simulink model "stateEstimator"  (R2018a)
settings: Solver=VariableStepAuto  StartTime=0.0  StopTime=10.0  RelTol=1e-3
undefined symbols (not defined in the file): SkywalkerX8
libraries: simulink_extras x5, sharedTrackingLibrary x2
settings Model: Creator=David  LastModifiedBy=David

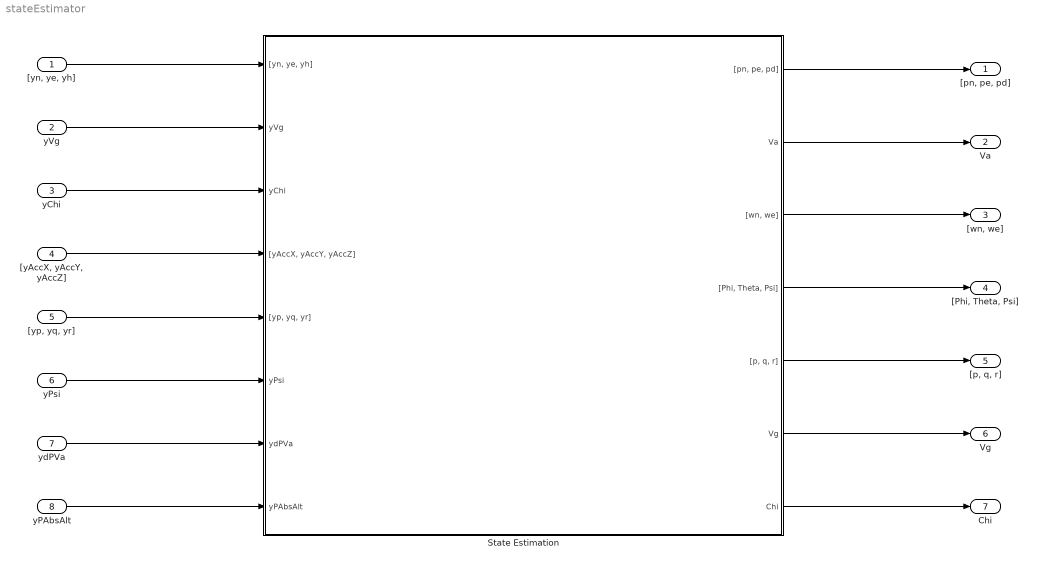
== system stateEstimator ==
  "[yn, ye, yh]" : Inport  PortDimensions=3
  yVg : Inport  Port=2  PortDimensions=3
  yChi : Inport  Port=3  PortDimensions=3
  "[yAccX, yAccY, yAccZ]" : Inport  Port=4  PortDimensions=3
  "[yp, yq, yr]" : Inport  Port=5  PortDimensions=3
  yPsi : Inport  Port=6  PortDimensions=3
  ydPVa : Inport  Port=7  PortDimensions=3
  yPAbsAlt : Inport  Port=8  PortDimensions=3
  State Estimation : Subsystem
      mask Display:
      | image('state_estimate.jpg', 'center')
      | 
      | port_label('input', 1, '[y_{GPS_N}, y_{GPS_E}, y_{GPS_h}] (m)', 'texMode', 'On')
      | port_label('input', 2, 'y_{GPS_{Vg}} (m/s)', 'texMode', 'On')
      | port_label('input', 3, 'y_{GPS_{\chi}} (rad)', 'texMode', 'On')
      | port_label('input', 4, '[y_{accel_x}, y_{accel_y}, y_{accel_z}] (m/s^2)', 'texMode', 'on')
      | port_label('input', 5, '[y_p, y_q, y_r] (rad/s)', 'texMode', 'on')
      | port_label('input', 6, 'y_{\psi} (rad)', 'texMode', 'on')
      | port_label('input', 7, 'y_{\DeltaP_{V_a}} (Pa)', 'texMode', 'on')
      | port_label('input', 8, 'y_{P_{abs}} (Pa)', 'texMode', 'on')
      | 
      | port_label('output', 1, '[p_N, p_E, p_D] (m)', 'texMode', 'On')
      | port_label('output', 2, 'V_a (m/s)', 'texMode', 'On')
      | port_label('output', 3, '[w_N, w_E] (m/s)', 'texMode', 'On')
      | port_label('output', 4, '[\phi, \theta, \psi] (rad)', 'texMode', 'on')
      | port_label('output', 5, '{\bf\omega_b} (rad/s)', 'texMode', 'on')
      | port_label('output', 6, 'V_g (m/s)', 'texMode', 'on')
      | port_label('output', 7, '\chi (rad)', 'texMode', 'on')
  "[pn, pe, pd]" : Outport
  Va : Outport  Port=2
  "[wn, we]" : Outport  Port=3
  "[Phi, Theta, Psi]" : Outport  Port=4
  "[p, q, r]" : Outport  Port=5
  Vg : Outport  Port=6
  Chi : Outport  Port=7
  wires:
  "[yn, ye, yh]"/1 -> State Estimation/1("[yn, ye, yh]")
  yVg/1 -> State Estimation/2(yVg)
  yChi/1 -> State Estimation/3(yChi)
  "[yAccX, yAccY, yAccZ]"/1 -> State Estimation/4("[yAccX, yAccY, yAccZ]")
  "[yp, yq, yr]"/1 -> State Estimation/5("[yp, yq, yr]")
  yPsi/1 -> State Estimation/6(yPsi)
  ydPVa/1 -> State Estimation/7(ydPVa)
  yPAbsAlt/1 -> State Estimation/8(yPAbsAlt)
  State Estimation/1("[pn, pe, pd]") -> "[pn, pe, pd]"/1
  State Estimation/2(Va) -> Va/1
  State Estimation/3("[wn, we]") -> "[wn, we]"/1
  State Estimation/4("[Phi, Theta, Psi]") -> "[Phi, Theta, Psi]"/1
  State Estimation/5("[p, q, r]") -> "[p, q, r]"/1
  State Estimation/6(Vg) -> Vg/1
  State Estimation/7(Chi) -> Chi/1

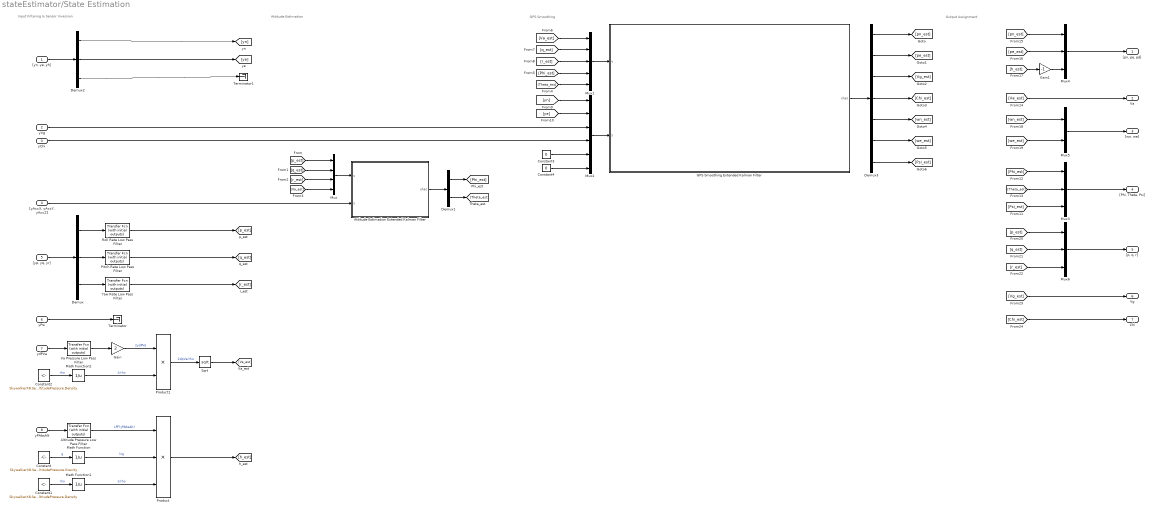
== system stateEstimator/State Estimation ==
  note: Output Assignment
  note: GPS Smoothing
  note: Attitude Estimation
  note: Input Filtering & Sensor Inversion
  "[yn, ye, yh]" : Inport  PortDimensions=3
  yVg : Inport  Port=2  PortDimensions=3
  yChi : Inport  Port=3  PortDimensions=3
  "[yAccX, yAccY, yAccZ]" : Inport  Port=4  PortDimensions=3
  "[yp, yq, yr]" : Inport  Port=5  PortDimensions=3
  yPsi : Inport  Port=6  PortDimensions=3
  ydPVa : Inport  Port=7  PortDimensions=3
  yPAbsAlt : Inport  Port=8  PortDimensions=3
  Altitude Pressure Low Pass Filter : simulink_extras/Additional Linear/Transfer Fcn (with initial outputs)  N=cell2mat(SkywalkerX8.Sensors.Filters.AltitudePressure.FilterTF.Numerator)  D=cell2mat(SkywalkerX8.Sensors.Filters.AltitudePressure.FilterTF.Denominator)  Y0=SkywalkerX8.Sensors.Filters.AltitudePressure.InitialCondition  U0=SkywalkerX8.Sensors.Filters.AltitudePressure.InitialCondition
  Attitude Estimation Extended Kalman Filter : Subsystem
      mask Display:
      | port_label('input', 1, '{\bf u} = [p, q, r, V_a]', 'texMode', 'On')
      | port_label('input', 2, '{\bf y} = [a_x, a_y, a_z]', 'texMode', 'On')
      | 
      | port_label('output', 1, '{\bf x_{est}} = [\Phi, \theta]', 'texMode', 'On')
  Constant : Constant  Value=SkywalkerX8.Sensors.StateEstimate.SensorInversion.AltitudePressure.Gravity
  Constant1 : Constant  Value=SkywalkerX8.Sensors.StateEstimate.SensorInversion.AltitudePressure.Density
  Constant2 : Constant  Value=SkywalkerX8.Sensors.StateEstimate.SensorInversion.AltitudePressure.Density
  Constant3 : Constant  Value=0
  Constant4 : Constant  Value=0
  Demux : Demux  Outputs=3
  Demux1 : Demux  Outputs=2
  Demux2 : Demux  Outputs=3
  Demux3 : Demux  Outputs=7
  GPS Smoothing Extended Kalman Filter : Subsystem
      mask Display:
      | port_label('input', 1, '{\bf u} = [V_a, q, r, \Phi, \theta]', 'texMode', 'On')
      | port_label('input', 2, '{\bf y} = [y_{GPS_N}, y_{GPS_E}, y_{GPS_{V_g}}, y_{GPS_\chi}, y_{GPS_{wind_N}}, y_{GPS_{wind_E}}]', 'texMode', 'On')
      | 
      | port_label('output', 1, '{\bf x_{est}} = [p_n, p_e, V_g, \chi, w_n, w_e, \psi]', 'texMode', 'On')
  Gain : Gain  Gain=2
  Gain1 : Gain  Gain=-1
  Math Function : Math  Operator=reciprocal  SaturateOnIntegerOverflow=on
  Math Function1 : Math  Operator=reciprocal  SaturateOnIntegerOverflow=on
  Math Function2 : Math  Operator=reciprocal  SaturateOnIntegerOverflow=on
  Mux : Mux
  Mux1 : Mux  Inputs=5
  Mux2 : Mux  Inputs=6
  Mux3 : Mux  Inputs=3
  Mux4 : Mux  Inputs=3
  Mux5 : Mux  Inputs=2
  Mux6 : Mux  Inputs=3
  Pitch Rate Low Pass Filter : simulink_extras/Additional Linear/Transfer Fcn (with initial outputs)  N=cell2mat(SkywalkerX8.Sensors.Filters.AngularRates.Pitch.FilterTF.Numerator)  D=cell2mat(SkywalkerX8.Sensors.Filters.AngularRates.Pitch.FilterTF.Denominator)  Y0=SkywalkerX8.Sensors.Filters.AngularRates.Pitch.InitialCondition  U0=SkywalkerX8.Sensors.Filters.AngularRates.Pitch.InitialCondition
  Product : Product  Inputs=3
  Product1 : Product
  Roll Rate Low Pass Filter : simulink_extras/Additional Linear/Transfer Fcn (with initial outputs)  N=cell2mat(SkywalkerX8.Sensors.Filters.AngularRates.Roll.FilterTF.Numerator)  D=cell2mat(SkywalkerX8.Sensors.Filters.AngularRates.Roll.FilterTF.Denominator)  Y0=SkywalkerX8.Sensors.Filters.AngularRates.Roll.InitialCondition  U0=SkywalkerX8.Sensors.Filters.AngularRates.Roll.InitialCondition
  Sqrt : Sqrt  SaturateOnIntegerOverflow=on
  Terminator : Terminator
  Terminator1 : Terminator
  Va Pressure Low Pass Filter : simulink_extras/Additional Linear/Transfer Fcn (with initial outputs)  N=cell2mat(SkywalkerX8.Sensors.Filters.AirspeedPressure.FilterTF.Numerator)  D=cell2mat(SkywalkerX8.Sensors.Filters.AirspeedPressure.FilterTF.Denominator)  Y0=SkywalkerX8.Sensors.Filters.AirspeedPressure.InitialCondition  U0=SkywalkerX8.Sensors.Filters.AirspeedPressure.InitialCondition
  Yaw Rate Low Pass Filter : simulink_extras/Additional Linear/Transfer Fcn (with initial outputs)  N=cell2mat(SkywalkerX8.Sensors.Filters.AngularRates.Yaw.FilterTF.Numerator)  D=cell2mat(SkywalkerX8.Sensors.Filters.AngularRates.Yaw.FilterTF.Denominator)  Y0=SkywalkerX8.Sensors.Filters.AngularRates.Yaw.InitialCondition  U0=SkywalkerX8.Sensors.Filters.AngularRates.Yaw.InitialCondition
  "[pn, pe, pd]" : Outport
  Va : Outport  Port=2
  "[wn, we]" : Outport  Port=3
  "[Phi, Theta, Psi]" : Outport  Port=4
  "[p, q, r]" : Outport  Port=5
  Vg : Outport  Port=6
  Chi : Outport  Port=7
  wires:
  [Phi_est] -> Mux1/4
  Math Function1/1 -> Product/3  "1/rho"
  [ye] -> Mux2/2
  Sqrt/1 -> [Va_est]
  Demux/2 -> Pitch Rate Low Pass Filter/1
  [r_est] -> Mux/3
  Math Function2/1 -> Product1/2  "1/rho"
  yChi/1 -> Mux2/4
  Demux2/3 -> Terminator1/1
  Mux4/1 -> "[pn, pe, pd]"/1
  Mux6/1 -> "[p, q, r]"/1
  [r_est] -> Mux1/3
  Constant3/1 -> Mux2/5
  Constant2/1 -> Math Function2/1  "rho"
  Demux3/4 -> [Chi_est]
  Demux3/3 -> [Vg_est]
  Gain1/1 -> Mux4/3
  Math Function/1 -> Product/2  "1/g"
  [h_est] -> Gain1/1
  [we_est] -> Mux5/2
  "[yp, yq, yr]"/1 -> Demux/1
  [Theta_est] -> Mux1/5
  Demux3/7 -> [Psi_est]
  Mux2/1 -> GPS Smoothing Extended Kalman Filter/2(y)
  Constant4/1 -> Mux2/6
  [r_est] -> Mux6/3
  Mux/1 -> Attitude Estimation Extended Kalman Filter/1(u)
  [wn_est] -> Mux5/1
  Demux2/2 -> [ye]
  GPS Smoothing Extended Kalman Filter/1(xhat) -> Demux3/1
  Constant1/1 -> Math Function1/1  "rho"
  Demux2/1 -> [yn]
  Demux3/6 -> [we_est]
  [q_est] -> Mux6/2
  "[yAccX, yAccY, yAccZ]"/1 -> Attitude Estimation Extended Kalman Filter/2(y)
  Demux1/2 -> [Theta_est]
  Mux1/1 -> GPS Smoothing Extended Kalman Filter/1(u)
  Demux3/5 -> [wn_est]
  Attitude Estimation Extended Kalman Filter/1(xhat) -> Demux1/1
  Gain/1 -> Product1/1  "2ydPVa"
  Constant/1 -> Math Function/1  "g"
  [p_est] -> Mux/1
  yVg/1 -> Mux2/3
  Altitude Pressure Low Pass Filter/1 -> Product/1  "LPF(yPAbsAlt)"
  [Chi_est] -> Chi/1
  yPsi/1 -> Terminator/1
  [q_est] -> Mux1/2
  Demux3/1 -> [pn_est]
  [Va_est] -> Mux1/1
  [Theta_est] -> Mux3/2
  Va Pressure Low Pass Filter/1 -> Gain/1
  [q_est] -> Mux/2
  Product1/1 -> Sqrt/1  "2dpVa/rho"
  Yaw Rate Low Pass Filter/1 -> [r_est]
  Product/1 -> [h_est]
  [Va_est] -> Mux/4
  ydPVa/1 -> Va Pressure Low Pass Filter/1
  [Psi_est] -> Mux3/3
  Pitch Rate Low Pass Filter/1 -> [q_est]
  Demux/1 -> Roll Rate Low Pass Filter/1
  yPAbsAlt/1 -> Altitude Pressure Low Pass Filter/1
  Demux/3 -> Yaw Rate Low Pass Filter/1
  [pn_est] -> Mux4/1
  [p_est] -> Mux6/1
  Demux3/2 -> [pe_est]
  Demux1/1 -> [Phi_est]
  Roll Rate Low Pass Filter/1 -> [p_est]
  [Vg_est] -> Vg/1
  "[yn, ye, yh]"/1 -> Demux2/1
  [pe_est] -> Mux4/2
  [Phi_est] -> Mux3/1
  Mux3/1 -> "[Phi, Theta, Psi]"/1
  Mux5/1 -> "[wn, we]"/1
  [Va_est] -> Va/1
  [yn] -> Mux2/1

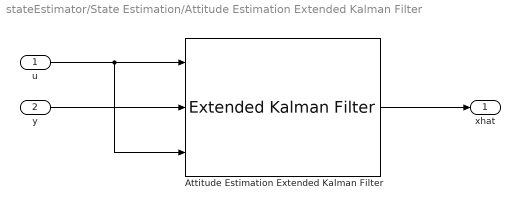
== system stateEstimator/State Estimation/Attitude Estimation Extended Kalman Filter ==
  u : Inport
  y : Inport  Port=2
  Attitude Estimation Extended Kalman Filter : sharedTrackingLibrary/Extended Kalman Filter  StateTransitionFcn=attitudeTransitionEstimate  HasStateTransitionJacobianFcn=on  StateTransitionJacobianFcn=attitudeTransitionEstimate_Jacobian  HasAdditiveProcessNoise=Additive  ProcessNoise=SkywalkerX8.Sensors.EKF.Attitude.StateCovarianceMatrix  HasTimeVaryingProcessNoise=off  HasStateTransitionFcnExtraArgument=1  InitialState=SkywalkerX8.Sensors.EKF.Attitude.InitialState  InitialStateCovariance=SkywalkerX8.Sensors.EKF.Attitude.InitialStateCovarianceMatrix  MeasurementFcn1=accelerometerMeasurementEstimate  HasMeasurementJacobianFcn1=on  MeasurementJacobianFcn1=accelerometerMeasurementEstimate_Jacobian  HasMeasurementEnablePort1=off  HasAdditiveMeasurementNoise1=Additive  MeasurementNoise1=SkywalkerX8.Sensors.EKF.Attitude.MeasurementCovarianceMatrix  HasTimeVaryingMeasurementNoise1=off  HasMeasurementFcnExtraArgument1=1  MeasurementFcn2=myMeasurementFcn  HasMeasurementJacobianFcn2=off  HasMeasurementEnablePort2=off  HasAdditiveMeasurementNoise2=Additive  MeasurementNoise2=1  HasTimeVaryingMeasurementNoise2=off  HasMeasurementFcnExtraArgument2=0  MeasurementFcn3=myMeasurementFcn  HasMeasurementJacobianFcn3=off  HasMeasurementEnablePort3=off  HasAdditiveMeasurementNoise3=Additive  MeasurementNoise3=1  HasTimeVaryingMeasurementNoise3=off  HasMeasurementFcnExtraArgument3=0  MeasurementFcn4=myMeasurementFcn  HasMeasurementJacobianFcn4=off  HasMeasurementEnablePort4=off  HasAdditiveMeasurementNoise4=Additive  MeasurementNoise4=1  HasTimeVaryingMeasurementNoise4=off  HasMeasurementFcnExtraArgument4=0  MeasurementFcn5=myMeasurementFcn  HasMeasurementJacobianFcn5=off  HasMeasurementEnablePort5=off  HasAdditiveMeasurementNoise5=Additive  MeasurementNoise5=1  HasTimeVaryingMeasurementNoise5=off  HasMeasurementFcnExtraArgument5=0  EnableMultirate=on  StateTransitionFcnSampleTime=SkywalkerX8.Sensors.EKF.Attitude.StateTransitionSampleTime  MeasurementFcn1SampleTime=SkywalkerX8.Sensors.EKF.Attitude.MeasurementSampleTime  MeasurementFcn2SampleTime=1  MeasurementFcn3SampleTime=1  MeasurementFcn4SampleTime=1  MeasurementFcn5SampleTime=1  UseCurrentEstimator=on  OutputStateCovariance=off  DataType=double  SampleTime=SkywalkerX8.Sensors.EKF.Attitude.SampleTime  NumberOfMeasurements=1
      settings: SourceProductName=Control System Toolbox  SourceProductBaseCode=CT
  xhat : Outport
  wires:
  y/1 -> Attitude Estimation Extended Kalman Filter/2
  u/1 -> Attitude Estimation Extended Kalman Filter/3, Attitude Estimation Extended Kalman Filter/1
  Attitude Estimation Extended Kalman Filter/1 -> xhat/1

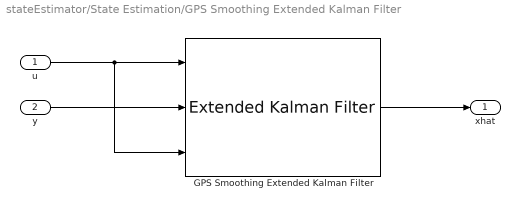
== system stateEstimator/State Estimation/GPS Smoothing Extended Kalman Filter ==
  u : Inport
  y : Inport  Port=2
  GPS Smoothing Extended Kalman Filter : sharedTrackingLibrary/Extended Kalman Filter  StateTransitionFcn=GPSSmoothingTransitionEstimate  HasStateTransitionJacobianFcn=on  StateTransitionJacobianFcn=GPSSmoothingTransitionEstimate_Jacobian  HasAdditiveProcessNoise=Additive  ProcessNoise=SkywalkerX8.Sensors.EKF.GPSSmoothing.StateCovarianceMatrix  HasTimeVaryingProcessNoise=off  HasStateTransitionFcnExtraArgument=1  InitialState=SkywalkerX8.Sensors.EKF.GPSSmoothing.InitialState  InitialStateCovariance=SkywalkerX8.Sensors.EKF.GPSSmoothing.InitialStateCovarianceMatrix  MeasurementFcn1=GPSSmoothingMeasurementEstimate  HasMeasurementJacobianFcn1=on  MeasurementJacobianFcn1=GPSSmoothingMeasurementEstimate_Jacobian  HasMeasurementEnablePort1=off  HasAdditiveMeasurementNoise1=Additive  MeasurementNoise1=SkywalkerX8.Sensors.EKF.GPSSmoothing.MeasurementCovarianceMatrix  HasTimeVaryingMeasurementNoise1=off  HasMeasurementFcnExtraArgument1=1  MeasurementFcn2=myMeasurementFcn  HasMeasurementJacobianFcn2=off  HasMeasurementEnablePort2=off  HasAdditiveMeasurementNoise2=Additive  MeasurementNoise2=1  HasTimeVaryingMeasurementNoise2=off  HasMeasurementFcnExtraArgument2=0  MeasurementFcn3=myMeasurementFcn  HasMeasurementJacobianFcn3=off  HasMeasurementEnablePort3=off  HasAdditiveMeasurementNoise3=Additive  MeasurementNoise3=1  HasTimeVaryingMeasurementNoise3=off  HasMeasurementFcnExtraArgument3=0  MeasurementFcn4=myMeasurementFcn  HasMeasurementJacobianFcn4=off  HasMeasurementEnablePort4=off  HasAdditiveMeasurementNoise4=Additive  MeasurementNoise4=1  HasTimeVaryingMeasurementNoise4=off  HasMeasurementFcnExtraArgument4=0  MeasurementFcn5=myMeasurementFcn  HasMeasurementJacobianFcn5=off  HasMeasurementEnablePort5=off  HasAdditiveMeasurementNoise5=Additive  MeasurementNoise5=1  HasTimeVaryingMeasurementNoise5=off  HasMeasurementFcnExtraArgument5=0  EnableMultirate=on  StateTransitionFcnSampleTime=SkywalkerX8.Sensors.EKF.GPSSmoothing.StateTransitionSampleTime  MeasurementFcn1SampleTime=SkywalkerX8.Sensors.EKF.GPSSmoothing.MeasurementSampleTime  MeasurementFcn2SampleTime=1  MeasurementFcn3SampleTime=1  MeasurementFcn4SampleTime=1  MeasurementFcn5SampleTime=1  UseCurrentEstimator=on  OutputStateCovariance=off  DataType=double  NumberOfMeasurements=1
      settings: SourceProductName=Control System Toolbox  SourceProductBaseCode=CT
  xhat : Outport
  wires:
  y/1 -> GPS Smoothing Extended Kalman Filter/2
  u/1 -> GPS Smoothing Extended Kalman Filter/3, GPS Smoothing Extended Kalman Filter/1
  GPS Smoothing Extended Kalman Filter/1 -> xhat/1
